simulink model "SixWheelModel"  (R2020b)
settings: Solver=VariableStepAuto  StartTime=0.0  StopTime=10.0  RelTol=1e-6
model workspace (MATLAB code in the model file):
  | EditVars
undefined symbols (not defined in the file or in its folder): incline, magicCoefficients, pwmVolt, rotorInertia, roverMass, wheelMass, wheelRadius
libraries: ee_lib x24, fl_lib x20, sdl_lib x13, nesl_utility x11
settings Model: Creator=lemck  LastModifiedBy=lemck

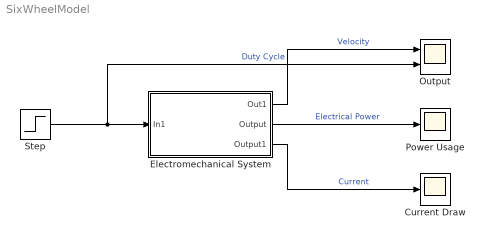
== system SixWheelModel ==
  Current Draw : Scope
  Electromechanical System : Subsystem
  Output : Scope  NumInputPorts=2
  Power Usage : Scope
  Step : Step  After=0.3  SampleTime=0
  wires:
  Electromechanical System/1(Out1) -> Output/1  "Velocity"
  Electromechanical System/2(Output) -> Power Usage/1  "Electrical Power"
  Electromechanical System/3(Output1) -> Current Draw/1  "Current"
  Step/1 -> Output/2, Electromechanical System/1(In1)  "Duty Cycle"

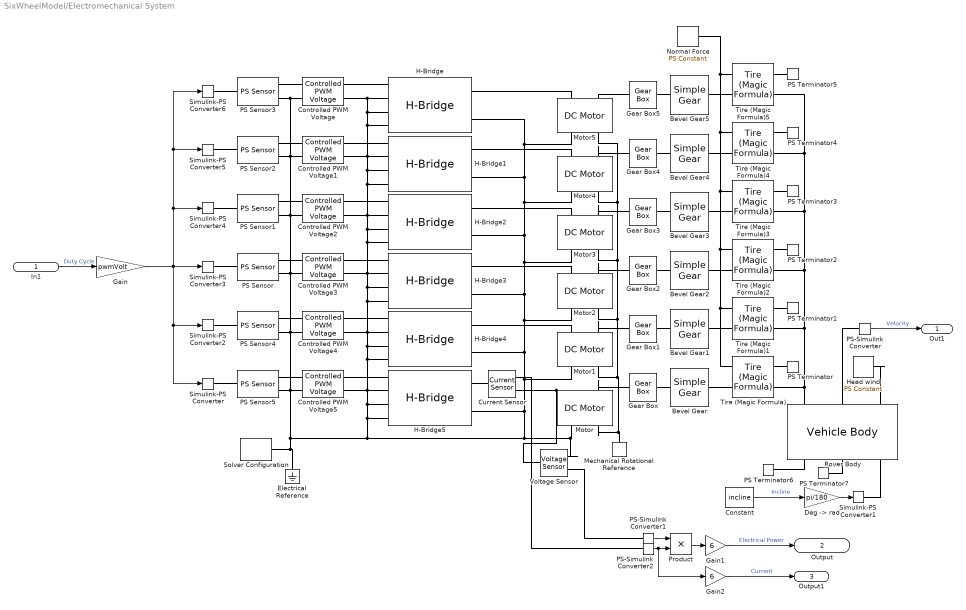
== system SixWheelModel/Electromechanical System ==
  In1 : Inport
   Gear Box{,1..5} (6 alike) : fl_lib/Mechanical/Mechanisms/Gear Box  ratio=gbRatio  t_in_specify=off  t_in_priority=None  t_in=0 N*m  t_in_nominal_specify=off  t_in_nominal_unit=N*m  t_in_nominal_value=1  t_out_specify=off  t_out_priority=None  t_out=0 N*m  t_out_nominal_specify=off  t_out_nominal_unit=N*m  t_out_nominal_value=1
  Bevel Gear{,1..5} (6 alike) : sdl_lib/Gears/Simple Gear  ratio=bevelRatio  rotation_direction=sdl.enum.shaftOutputDirection.same  friction_model=sdl.enum.gear_efficiencies_load.constant  mu_visc=[0, 0] N*m/(rad/s)  T_noload=0.1 N*m  T_nom=5 N*m  efficiency_nom=0.8  efficiency=bevelEfficiency  temperature_TLU=[280, 300, 320] K  load_TLU=[1, 5, 10] N*m  efficiency_TLU=[.95, .9, .85]  efficiency_TLU2=[.85, .8, .75; .95, .9, .85; .85, .8, .7]  w_thr=0.01 rad/s  pwr_thr=0.001 W  thermal_mass=50 J/K  enable_faults=simscape.enum.onoff.off  efficiency_fault=0.05  external_fault=simscape.enum.onoff.off  temporal_fault=simscape.enum.onoff.off  fault_time=5 s  fault_angles=pi / 12 rad  report_fault=simscape.enum.assert.action.none  temperature_specify=off  temperature_priority=High  temperature=300 K  temperature_nominal_specify=off  temperature_nominal_unit=K  temperature_nominal_value=1
  Constant : Constant  Value=incline
  Controlled PWM Voltage{,1..5} (6 alike) : ee_lib/Integrated Circuits/Controlled PWM Voltage  F=pwmFreq Hz  TD=0 s  pulse_width_offset=0 s  pulse_min=0 s  Vmin=0 V  Vmax=pwmVolt V  Vm=pwmVolt V  pwm_or_av=2  event_type=1  sample_time=1e-6 s  u_min=0  u_max=1
  Current Sensor : fl_lib/Electrical/Electrical Sensors/Current Sensor
  "Deg -> rad" : Gain  Gain=pi/180
  Electrical Reference : fl_lib/Electrical/Electrical Elements/Electrical Reference
  Gain : Gain  Gain=pwmVolt
  Gain1 : Gain  Gain=6
  Gain2 : Gain  Gain=6
  H-Bridge{,1..5} (6 alike) : ee_lib/Semiconductors & Converters/Converters/H-Bridge  supply_ports=ee.enum.supply_ports.hidesupply  Venable=pwmVolt/2 V  Vmax=pwmVolt V  Vreverse=pwmVolt/2 V  Vbrake=pwmVolt/2 V  Vm=ratedVolt V  pwm_or_av=ee.enum.pwm_or_av.averaged  regenerative_braking_mode=ee.enum.converters.regenerative_braking_mode.depends_on_rev  discontinuous=ee.enum.current_profile.continuous  freewheeling_mode=ee.enum.converters.freewheeling_mode.one_switch_one_diode  Ron=1e-6 Ohm  Don=0.05 Ohm  Goff=1e-6 S  Rload=10 Ohm  Lload=1e-5 H  F=10 kHz  thermal_mass=100 J/K  initial_temperature=298.15 K  Ron2=0.1 Ohm  Don2=0.05 Ohm  Tmeas=298.15 K  Tmeas2=398.15 K
  Head wind : fl_lib/Physical Signals/Sources/PS Constant  constant=headWindSpeed m/s
  Mechanical Rotational Reference : fl_lib/Mechanical/Rotational Elements/Mechanical Rotational Reference
  Motor : ee_lib/Electromechanical/Brushed Motors/DC Motor  field_option=ee.enum.field_option.pm  Rf=100 Ohm  Lf=1 H  Laf=0.15 H  If0=0 A  parameterization=ee.enum.dcparam_option.torque_speed  Ra=3.9 Ohm  La=armInductance H  emf_or_torque=ee.enum.emf_or_torque.kv  Kv=0.072e-3 V/rpm  Ki=6.876e-4 N*m/A  T_stall=stallTorque N*m  w_max=freeSpeed rpm  w_rated=15000 rpm  P_rated=149 W  V_rated=ratedVolt V  J=rotorInertia g*cm^2  lam_param=ee.enum.lam_param.current  lam=0 N*m/(rad/s)  i_noload=currentMin A  V_i_noload=ratedVolt V  speed0=0 rpm  enable_fault_armature=ee.enum.faults.faultEnable.no  rev_faulted=1 / 3  G_faulted_armature=1e-5 S  fault_trigger_armature=ee.enum.faults.faultTrigger.temporal  t_fault_armature=1 s  max_permissible_current_armature=inf A  t_fail_on_current_armature=1 s  enable_fault_field=ee.enum.faults.faultEnable.no  G_faulted_field=1e-5 S  fault_trigger_field=ee.enum.faults.faultTrigger.temporal  t_fault_field=1 s  max_permissible_current_field=inf A  t_fail_on_current_field=1 s  fault_action=ee.enum.faults.faultAction.none  alpha=3.93e-3 1/K  Tmeas=25 degC  thermal_mass=100 J/K  initial_temperature=25 degC
  Motor{1..5} (5 alike) : ee_lib/Electromechanical/Brushed Motors/DC Motor  field_option=ee.enum.field_option.pm  Rf=100 Ohm  Lf=1 H  Laf=0.15 H  If0=0 A  parameterization=ee.enum.dcparam_option.torque_speed  Ra=3.9 Ohm  La=armInductance H  emf_or_torque=ee.enum.emf_or_torque.kv  Kv=0.072e-3 V/rpm  Ki=6.876e-4 N*m/A  T_stall=stallTorque N*m  w_max=freeSpeed rpm  w_rated=15000 rpm  P_rated=0.08 W  V_rated=ratedVolt V  J=rotorInertia g*cm^2  lam_param=ee.enum.lam_param.current  lam=0 N*m/(rad/s)  i_noload=currentMin A  V_i_noload=ratedVolt V  speed0=0 rpm  enable_fault_armature=ee.enum.faults.faultEnable.no  rev_faulted=1 / 3  G_faulted_armature=1e-5 S  fault_trigger_armature=ee.enum.faults.faultTrigger.temporal  t_fault_armature=1 s  max_permissible_current_armature=inf A  t_fail_on_current_armature=1 s  enable_fault_field=ee.enum.faults.faultEnable.no  G_faulted_field=1e-5 S  fault_trigger_field=ee.enum.faults.faultTrigger.temporal  t_fault_field=1 s  max_permissible_current_field=inf A  t_fail_on_current_field=1 s  fault_action=ee.enum.faults.faultAction.none  alpha=3.93e-3 1/K  Tmeas=25 degC  thermal_mass=100 J/K  initial_temperature=25 degC
  Normal Force : fl_lib/Physical Signals/Sources/PS Constant  constant=roverMass*9.81/6 N
  PS Sensor{,1..5} (6 alike) : ee_lib/Sensors & Transducers/PS Sensor  op_type=1  A=1  B=0  Ymax=inf  Ymin=0
      settings: SourceProductBaseCode=PS  InternalSimscapePortConfiguration="{\"Bottom\":[],\"Left\":[{\"id\":\"U\",\"label\":\"U\",\"type\":\"input\"}],\"Right\":[{\"id\":\"p\",\"label\":\"+\",\"type\":\"foundation.electrical.electrical\"},{\"id\":\"n\",\"label\":\"-\",\"type\":\"foundation.electrical.electrical\"}],\"Top\":[]}"
  PS Terminator{,1..7} (8 alike) : fl_lib/Physical Signals/Sinks/PS Terminator
  PS-Simulink Converter : nesl_utility/PS-Simulink Converter  PhysicalDomain=network_engine_domain  SubClassName=ps_output  LeftPortType=input  RightPortType=output  PseudoPeriodic=off  Frequencies=[]  Unit=inherit  AffineConversion=off
  PS-Simulink Converter1 : nesl_utility/PS-Simulink Converter  PhysicalDomain=network_engine_domain  SubClassName=ps_output  LeftPortType=input  RightPortType=output  PseudoPeriodic=off  Frequencies=[]  Unit=inherit  AffineConversion=off
  PS-Simulink Converter2 : nesl_utility/PS-Simulink Converter  PhysicalDomain=network_engine_domain  SubClassName=ps_output  LeftPortType=input  RightPortType=output  PseudoPeriodic=off  Frequencies=[]  Unit=inherit  AffineConversion=off
  Product : Product
  Rover Body : sdl_lib/Tires & Vehicles/Vehicle Body  mass=roverMass kg  n_w=2  x_f=1.4 m  x_r=1.6 m  y_c=0.5 m  mass_var=simscape.enum.onoff.off  model_pitch=simscape.enum.onoff.off  inertia=4000 kg*m^2  suspension_model=sdl.enum.linearTLU.linear  k_f=1e4 N/m  b_f=1e4 N/(m/s)  k_r=1e4 N/m  b_r=1e4 N/(m/s)  k_f_TLU=[-2000, -1000, 0, 1000, 2000] N  x_f_TLU=[-.4, -.2, 0, .2, .4] m  b_f_TLU=[-200, -100, 0, 100, 200] N  v_f_TLU=[-4, -2, 0, 2, 4] m/s  k_r_TLU=[-2000, -1000, 0, 1000, 2000] N  x_r_TLU=[-.4, -.2, 0, .2, .4] m  b_r_TLU=[-200, -100, 0, 100, 200] N  v_r_TLU=[-4, -2, 0, 2, 4] m/s  interp_method=simscape.enum.interpolation.linear  extrap_method=simscape.enum.extrapolation.linear  model_hardstop=simscape.enum.onoff.off  upper_bound_f=.25 m  lower_bound_f=-.25 m  stop_k_f=1e6 N/m  stop_b_f=150 N/(m/s)  upper_bound_r=.25 m  lower_bound_r=-.25 m  stop_k_r=1e6 N/m  stop_b_r=150 N/(m/s)  initial_pitch=0 rad  initial_pitch_rate=0 rad/s  g=9.81 m/s^2  liftoff_warning=simscape.enum.onoff.off  area=roverFrontalArea m^2  Cd=roverDragConst  rho=1.18 kg/m^3  v_specify=off  v_priority=High  v=0 m/s  v_nominal_specify=off  v_nominal_unit=m/s  v_nominal_value=1
  Simulink-PS Converter{,2..6} (6 alike) : nesl_utility/Simulink-PS Converter  PhysicalDomain=network_engine_domain  SubClassName=ps_input  LeftPortType=input  RightPortType=output  PseudoPeriodic=off  Frequencies=[]  NoiseDistribution=none  NoiseParameters=[]  Unit=1  AffineConversion=off  FilteringAndDerivatives=provide  SimscapeFilterOrder=1  InputFilterTimeConstant=0.001  UdotUserProvided=0
  Simulink-PS Converter1 : nesl_utility/Simulink-PS Converter  PhysicalDomain=network_engine_domain  SubClassName=ps_input  LeftPortType=input  RightPortType=output  PseudoPeriodic=off  Frequencies=[]  NoiseDistribution=none  NoiseParameters=[]  Unit=rad  AffineConversion=off  FilteringAndDerivatives=provide  SimscapeFilterOrder=1  InputFilterTimeConstant=0.001  UdotUserProvided=0
  Solver Configuration : nesl_utility/Solver Configuration  PhysicalDomain=network_engine_domain  SubClassName=solver  LeftPortType=input  RightPortType=generic  Tones=[]  Harmonics=[]  SimulateNoise=off  Profile=off  UseLocalSampling=off  EnableSwitchedLinearOptims=on  FrequencyDomain=off  UseCCode=off  RelTol=0.001  AbsTol=1e-06  MinStep=1e-09  ToWorkspace=off  RevertToSquareIcSolve=off  NumHomotopyIterations=100  PhasorMode=off  PhasorModeNumHarmonics=1  DoDC=off  ResidualTolerance=1e-09  UseLocalSolver=off  LocalSolverChoice=NE_BACKWARD_EULER_ADVANCER  LocalSolverSampleTime=0.001  DoFixedCost=off  MaxNonlinIter=3  MaxModeIter=2  ComputeImpulses=off  ImpulseIterations=2  LinearAlgebra=auto  EquationFormulation=NE_TIME_EF  DelaysMemoryBudget=1024  AutomaticFiltering=on  FilteringTimeConstant=0.001  PartitionStorageMethod=AS_NEEDED  PartitionMemoryBudget=1024  PartitionMethod=ROBUST
  Tire (Magic Formula){,1..4} (5 alike) : sdl_lib/Tires & Vehicles/Tire (Magic Formula)  parameterization=sdl.enum.magic_tire_model.constant  F_z1=3000 N  F_x1=3500 N  kappa1=10  B_m=magicCoefficients(1)  C_m=magicCoefficients(2)  D_m=magicCoefficients(3)  E_m=magicCoefficients(4)  fz0=4000 N  p_Cx=1.685  p_Dx=[1.21, -.037]  p_Ex=[.344, .095, -.02, 0]  p_Kx=[21.51, -.163, .245]  p_Hx=[-.002, .002]  p_Vx=[0, 0]  v_tr_thr=0.1 m/s  r_e=wheelRadius m  model_compliance=0  stiffness=1e6 N/m  damping=1000 N/(m/s)  model_inertia=1  inertia=wheelMass*wheelRadius^2 kg*m^2  initial_velocity=0 rad/s  model_resistance=0  resistance_model=1  coeff=0.015  p_tire=250e3 Pa  alpha=-0.003  beta=0.97  coeff_a=84e-4  coeff_b=6.2e-4 s/m  coeff_c=1.6e-4 s^2/m^2  v_thr=0.001 m/s
  Tire (Magic Formula)5 : sdl_lib/Tires & Vehicles/Tire (Magic Formula)  parameterization=sdl.enum.magic_tire_model.constant  F_z1=3000 N  F_x1=3500 N  kappa1=10  B_m=magicCoefficients(1)  C_m=magicCoefficients(2)  D_m=magicCoefficients(3)  E_m=magicCoefficients(4)  fz0=4000 N  p_Cx=1.685  p_Dx=[1.21, -.037]  p_Ex=[.344, .095, -.02, 0]  p_Kx=[21.51, -.163, .245]  p_Hx=[-.002, .002]  p_Vx=[0, 0]  v_tr_thr=0.1 m/s  r_e=wheelRadius m  model_compliance=0  stiffness=1e6 N/m  damping=1000 N/(m/s)  model_inertia=1  inertia=0.5*wheelMass*wheelRadius^2 kg*m^2  initial_velocity=0 rad/s  model_resistance=0  resistance_model=1  coeff=0.015  p_tire=250e3 Pa  alpha=-0.003  beta=0.97  coeff_a=84e-4  coeff_b=6.2e-4 s/m  coeff_c=1.6e-4 s^2/m^2  v_thr=0.001 m/s
  Voltage Sensor : fl_lib/Electrical/Electrical Sensors/Voltage Sensor
  Out1 : Outport
  Output : Outport  Port=2
  Output1 : Outport  Port=3
  wires:
  PS-Simulink Converter/1 -> Out1/1  "Velocity"
  "Deg -> rad"/1 -> Simulink-PS Converter1/1
  Constant/1 -> "Deg -> rad"/1  "Incline"
  In1/1 -> Gain/1  "Duty Cycle"
  Product/1 -> Gain1/1
  Gain1/1 -> Output/1  "Electrical Power"
  Gain2/1 -> Output1/1  "Current"
  Gain/1 -> Simulink-PS Converter/1, Simulink-PS Converter2/1, Simulink-PS Converter3/1, Simulink-PS Converter4/1, Simulink-PS Converter5/1, Simulink-PS Converter6/1
  PS-Simulink Converter2/1 -> Gain2/1, Product/2
  PS-Simulink Converter1/1 -> Product/1
  connections:
  Rover Body/RConn3 -- Simulink-PS Converter1/RConn1
  Tire (Magic Formula)/RConn2 -- Tire (Magic Formula)5/RConn2 -- Tire (Magic Formula)4/RConn2 -- Tire (Magic Formula)3/RConn2 -- Tire (Magic Formula)2/RConn2 -- Tire (Magic Formula)1/RConn2 -- Rover Body/LConn1
  Tire (Magic Formula)/RConn1 -- PS Terminator/LConn1
  Tire (Magic Formula)/LConn1 -- Tire (Magic Formula)1/LConn1 -- Tire (Magic Formula)2/LConn1 -- Tire (Magic Formula)3/LConn1 -- Tire (Magic Formula)4/LConn1 -- Tire (Magic Formula)5/LConn1 -- Normal Force/RConn1
  Bevel Gear/LConn1 -- " Gear Box"/RConn1
  Bevel Gear/RConn1 -- Tire (Magic Formula)/LConn2
  PS-Simulink Converter/LConn1 -- Rover Body/LConn2
  Bevel Gear1/RConn1 -- Tire (Magic Formula)1/LConn2
  Tire (Magic Formula)1/RConn1 -- PS Terminator1/LConn1
  Bevel Gear1/LConn1 -- " Gear Box1"/RConn1
  Bevel Gear2/RConn1 -- Tire (Magic Formula)2/LConn2
  Tire (Magic Formula)2/RConn1 -- PS Terminator2/LConn1
  Bevel Gear2/LConn1 -- " Gear Box2"/RConn1
  Bevel Gear3/RConn1 -- Tire (Magic Formula)3/LConn2
  Tire (Magic Formula)3/RConn1 -- PS Terminator3/LConn1
  Bevel Gear3/LConn1 -- " Gear Box3"/RConn1
  Bevel Gear4/LConn1 -- " Gear Box4"/RConn1
  Bevel Gear4/RConn1 -- Tire (Magic Formula)4/LConn2
  Tire (Magic Formula)4/RConn1 -- PS Terminator4/LConn1
  Bevel Gear5/LConn1 -- " Gear Box5"/RConn1
  Bevel Gear5/RConn1 -- Tire (Magic Formula)5/LConn2
  Tire (Magic Formula)5/RConn1 -- PS Terminator5/LConn1
  Head wind/RConn1 -- Rover Body/LConn3
  Motor/LConn2 -- " Gear Box"/LConn1
  Motor1/LConn2 -- " Gear Box1"/LConn1
  Motor/RConn2 -- Motor5/RConn2 -- Motor4/RConn2 -- Motor3/RConn2 -- Motor2/RConn2 -- Motor1/RConn2 -- Mechanical Rotational Reference/LConn1
  Motor2/LConn2 -- " Gear Box2"/LConn1
  Motor3/LConn2 -- " Gear Box3"/LConn1
  Motor4/LConn2 -- " Gear Box4"/LConn1
  " Gear Box5"/LConn1 -- Motor5/LConn2
  Motor/RConn1 -- Voltage Sensor/RConn2 -- H-Bridge5/LConn4 -- H-Bridge5/LConn3 -- H-Bridge5/LConn2 -- Controlled PWM Voltage5/RConn2 -- H-Bridge4/LConn3 -- H-Bridge4/LConn2 -- Controlled PWM Voltage4/RConn2 -- H-Bridge3/LConn4 -- H-Bridge3/LConn3 -- Controlled PWM Voltage3/RConn2 -- H-Bridge3/LConn2 -- H-Bridge2/LConn4 -- H-Bridge2/LConn3 -- H-Bridge2/LConn2 -- Controlled PWM Voltage2/RConn2 -- H-Bridge1/LConn4 -- H-Bridge1/LConn3 -- H-Bridge1/LConn2 -- H-Bridge/LConn4 -- H-Bridge/LConn3 -- Controlled PWM Voltage/RConn2 -- H-Bridge/LConn2 -- Controlled PWM Voltage1/RConn2 -- H-Bridge4/LConn4 -- PS Sensor3/RConn2 -- Controlled PWM Voltage/LConn2 -- PS Sensor2/RConn2 -- Controlled PWM Voltage1/LConn2 -- PS Sensor1/RConn2 -- Controlled PWM Voltage2/LConn2 -- PS Sensor/RConn2 -- Controlled PWM Voltage3/LConn2 -- Controlled PWM Voltage4/LConn2 -- PS Sensor4/RConn2 -- Controlled PWM Voltage5/LConn2 -- PS Sensor5/RConn2 -- Solver Configuration/RConn1 -- Electrical Reference/LConn1 -- H-Bridge5/RConn2 -- H-Bridge4/RConn2 -- Motor2/RConn1 -- Motor3/RConn1 -- Motor4/RConn1 -- Motor5/RConn1 -- H-Bridge/RConn2 -- H-Bridge1/RConn2 -- H-Bridge2/RConn2 -- H-Bridge3/RConn2 -- Motor1/RConn1
  Controlled PWM Voltage/RConn1 -- H-Bridge/LConn1
  Controlled PWM Voltage1/RConn1 -- H-Bridge1/LConn1
  Controlled PWM Voltage2/RConn1 -- H-Bridge2/LConn1
  Controlled PWM Voltage3/RConn1 -- H-Bridge3/LConn1
  Controlled PWM Voltage4/RConn1 -- H-Bridge4/LConn1
  Controlled PWM Voltage5/RConn1 -- H-Bridge5/LConn1
  PS Sensor/RConn1 -- Controlled PWM Voltage3/LConn1
  PS Sensor1/RConn1 -- Controlled PWM Voltage2/LConn1
  PS Sensor2/RConn1 -- Controlled PWM Voltage1/LConn1
  PS Sensor3/RConn1 -- Controlled PWM Voltage/LConn1
  PS Sensor4/RConn1 -- Controlled PWM Voltage4/LConn1
  PS Sensor5/RConn1 -- Controlled PWM Voltage5/LConn1
  Voltage Sensor/LConn1 -- Motor/LConn1 -- Current Sensor/RConn2
  Current Sensor/RConn1 -- PS-Simulink Converter2/LConn1
  Voltage Sensor/RConn1 -- PS-Simulink Converter1/LConn1
  Rover Body/RConn1 -- PS Terminator6/LConn1
  PS Terminator7/LConn1 -- Rover Body/RConn2
  Simulink-PS Converter/RConn1 -- PS Sensor5/LConn1
  Simulink-PS Converter2/RConn1 -- PS Sensor4/LConn1
  Simulink-PS Converter3/RConn1 -- PS Sensor/LConn1
  Simulink-PS Converter4/RConn1 -- PS Sensor1/LConn1
  Simulink-PS Converter5/RConn1 -- PS Sensor2/LConn1
  Simulink-PS Converter6/RConn1 -- PS Sensor3/LConn1
  H-Bridge3/RConn1 -- Motor2/LConn1
  H-Bridge4/RConn1 -- Motor1/LConn1
  H-Bridge2/RConn1 -- Motor3/LConn1
  H-Bridge1/RConn1 -- Motor4/LConn1
  Current Sensor/LConn1 -- H-Bridge5/RConn1
  H-Bridge/RConn1 -- Motor5/LConn1
